simulink model "R_model"  (R2018b)
settings: Solver=VariableStepAuto  StartTime=0.0  StopTime=10.0  RelTol=1e-3
model workspace (MAT data in the model file):
  b = 0.931
settings Model: Creator=rache  LastModifiedBy=rache

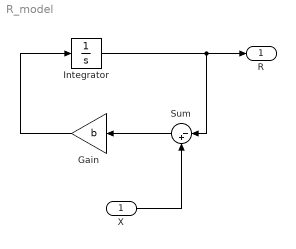
== system R_model ==
  X : Inport
  Gain : Gain  Gain=b
  Integrator : Integrator
  Sum : Sum  Inputs=|-+
  R : Outport
  wires:
  X/1 -> Sum/2
  Integrator/1 -> R/1, Sum/1
  Sum/1 -> Gain/1
  Gain/1 -> Integrator/1
